simulink model "psd_1"  (Simulink 4.00)
settings: Solver=FixedStepDiscrete  StartTime=0.0  StopTime=200  RelTol=1e-3
undefined symbols (not defined in the file or in its folder): get
libraries: dspbuff3 x1, dspddes3 x1, dspspect3 x1, dspstat3 x1, dspsnks3 x1
settings Model: LastModifiedBy=Administrator  BlockReductionOpt=off

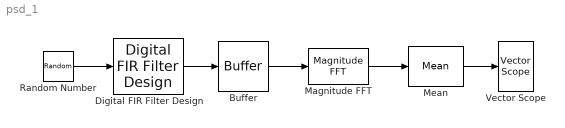
== system psd_1 ==
  Buffer : dspbuff3/Buffer  N=128  V=0  ic=0
  Digital FIR Filter Design : dspddes3/Digital FIR Filter Design  filttype=Lowpass  N=128  Wlo=0.4  Whi=0.6  W0=[.2 .5 .8]  g0=1  W1=[0 .2 .3 .6 .8 1]  gains=[1 .5 0 0 1 .5]  wintype=Hamming  Rs=10  Kbeta=5
  Magnitude FFT : dspspect3/Magnitude FFT  fftLenInherit=off  fftsize=256
  Mean : dspstat3/Mean  run=on  reset_popup=None
  Random Number : RandomNumber  Mean=0  Variance=1  Seed=0  SampleTime=0.1
  Vector Scope : dspsnks3/Vector Scope  ScopeProperties=off  Domain=Frequency  HorizSpan=1  DisplayProperties=off  AxisGrid=on  Memory=off  FrameNumber=on  AxisLegend=off  AxisZoom=off  OpenScopeAtSimStart=on  OpenScopeImmediately=off  FigPos=get(0,'defaultfigureposition')  AxisProperties=on  XUnits=Hertz  XRange=[0...Fs/2]  InheritXIncr=off  XIncr=0.1  XLabel=Time  YUnits=dB  YLabel=Amplitude  LineProperties=off
      settings: YMin=-10.2549892128968  YMax=24.3544697966047
  wires:
  Magnitude FFT/1 -> Mean/1
  Buffer/1 -> Magnitude FFT/1
  Mean/1 -> Vector Scope/1
  Digital FIR Filter Design/1 -> Buffer/1
  Random Number/1 -> Digital FIR Filter Design/1
